simulink model "auv_modell_camsim_vr"  (Simulink 7.0)
settings: Solver=ode45  StartTime=0.0  StopTime=1000  RelTol=1e-3
values from neighbouring files (symbols this model uses):
  eta0 = [-10 -7 7 0 0 0]'    [initauv.m]
undefined symbols (not defined in the file or in its folder): C_calc
libraries: marine_gnc x4, vrlib x2, simulink x1
settings Model: Creator=anderga  LastModifiedBy=anderga  BufferReuse=off
settings OptimizationCC: BlockReduction=off  InlineParams=on  BufferReuse=off

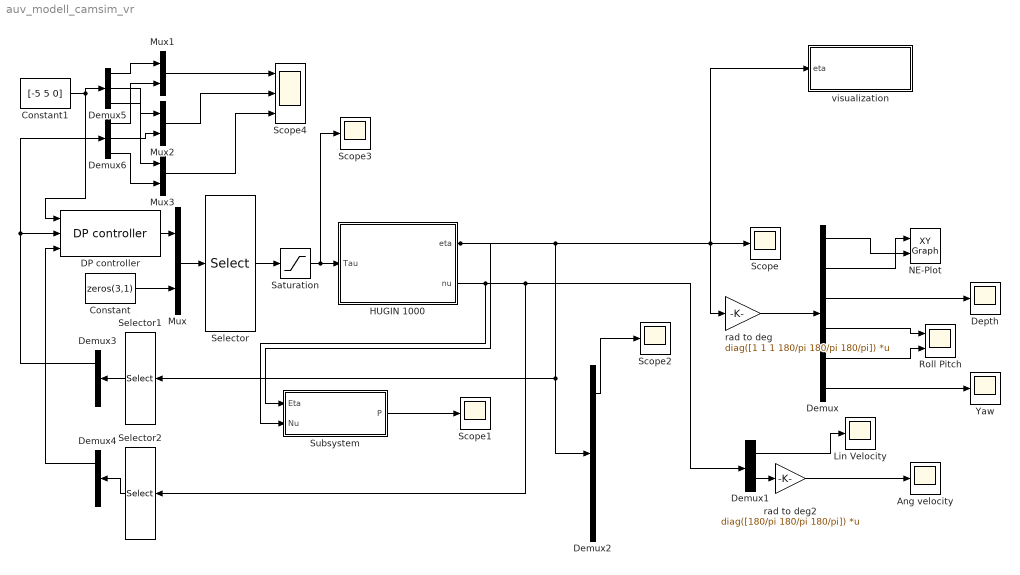
== system auv_modell_camsim_vr ==
  Ang velocity : Scope
      settings: YMin=-0.02  YMax=0.005  SaveName=ScopeData6
  Constant : Constant  Value=zeros(3,1)  OutDataType=sfix(16)  OutScaling=2^0
  Constant1 : Constant  Value=[-5 5 0]  OutDataType=sfix(16)  OutScaling=2^0
  DP controller : marine_gnc/Control/Dynamic  Positioning /DP controller  SystemSampleTime=-1  Kp=diag([230 300 1000])  Kd=diag([750 700 0])  Ki=diag([2 5 0])
  Demux : Demux  Outputs=6
  Demux1 : Demux  Outputs=2
  Demux2 : Demux  Outputs=3
  Demux3 : Demux  Orientation=left  Outputs=2
  Demux4 : Demux  Orientation=left  Outputs=2
  Demux5 : Demux  Outputs=3
  Demux6 : Demux  Outputs=3
  Depth : Scope
      settings: TimeRange=400  YMin=-20  YMax=10  SaveName=ScopeData4
  HUGIN 1000 : Subsystem  mask(HUGIN 1000 AUV){eta_0=eta0, nu_0=[0 0 0 0 0 0]}
      mask prompts: eta_0 "Initial Position [x y z phi theta psi]"; nu_0 "Initial speed [u v w p q r]"
      mask help:
      | The hydrodynamic model of Kongsberg Maritimes
      | AUV type HUGIN 1000.
      |
      | Implemented using
      |
      | eta_dot = J(eta)*nu
      | M*nu_dot + C(nu)*nu + D(nu)*nu + g(eta) = tau
      |
      | and the MMS toolbox from www.marinecybernetics.org
      mask init:
      | m = 1380;
      | xg = 0;
      | yg = 0;
      | zg = 0.0328;
      | Ix = 86.53;
      | Iy = 1247;
      | Iz = 1247;
      | 
      | Xu = -85.57;
      | Yv = -1092.9;
      | Yr = -84.1448;
      | Zw = -1092.9;
      | Zq = 84.1448;
      | Mq = -795.1686;
      | Nr = -795.1686;
      |     
      | M = [m-Xu   0       0       0       m*zg    -m*yg;
      |      0      m-Yv    0       -m*zg   0       m*xg-Yr;
      |      0      0       m-Zw    m*yg    -m*xg-Zq 0;
      |      0      -m*zg   m*yg    Ix      0        0;
      |      m*zg   0       -m*xg-Zq 0      Iy-Mq    0;
      |      -m*yg  m*xg-Yr 0       0       0       Iz-Nr];
  Lin Velocity : Scope
      settings: YMin=-6  YMax=9
  Mux{,1..3} (4 alike) : Mux  Inputs=2
  NE-Plot : simulink/Sinks/XY Graph  SystemSampleTime=-1  xmin=-100  xmax=220  ymin=-100  ymax=100  st=-1
  Roll Pitch : Scope  NumInputPorts=2
      settings: TimeRange=400  YMin=-0.01~-0.015  YMax=0.08~0.015  SaveName=ScopeData3
  Saturation : Saturate  UpperLimit=100  LowerLimit=-100  OutDataType=sfix(16)  OutScaling=2^0
  Scope{,1..3} (4 alike) : Scope
      Scope settings: YMin=-12.5  YMax=7.5
      Scope1 settings: YMin=-1  YMax=1  SaveName=ScopeData9
      Scope2 settings: YMin=-10  YMax=-10  SaveName=ScopeData10
      Scope3 settings: YMin=-100  YMax=100  SaveName=ScopeData11
  Scope4 : Scope  NumInputPorts=3
      settings: YMin=-10~-10~-2.25  YMax=5~12.5~0.75  SaveName=ScopeData12
  Selector : Selector  InputPortWidth=6  IndexOptions=Index vector (dialog)  Indices=[1 2 4 5 6 3]  OutputSizes=1
  Selector1 : Selector  Orientation=left  InputPortWidth=6  IndexOptions=Index vector (dialog)  Indices=[1 2 6 3 4 5]  OutputSizes=1
  Selector2 : Selector  Orientation=left  InputPortWidth=6  IndexOptions=Index vector (dialog)  Indices=[1 2 6 3 4 5]  OutputSizes=1
  Subsystem : Subsystem
  Yaw : Scope
      settings: TimeRange=100  YMin=-27.5  YMax=-7.5  SaveName=ScopeData2
  rad to deg : Gain  Gain=diag([1 1 1 180/pi 180/pi 180/pi])  Multiplication=Matrix(K*u)  ParameterDataType=sfix(16)  ParameterScaling=2^0  OutDataType=sfix(16)  OutScaling=2^0
  rad to deg2 : Gain  Gain=diag([180/pi 180/pi 180/pi])  Multiplication=Matrix(K*u)  ParameterDataType=sfix(16)  ParameterScaling=2^0  OutDataType=sfix(16)  OutScaling=2^0
  visualization : Subsystem
  wires:
  HUGIN 1000/1(eta) -> Subsystem/1(Eta), visualization/1(eta), rad to deg/1, Scope/1, Demux2/1, Selector1/1
  Demux/2 -> NE-Plot/1
  Demux/1 -> NE-Plot/2
  Demux/6 -> Yaw/1
  Demux/4 -> Roll Pitch/1
  Demux/5 -> Roll Pitch/2
  Demux/3 -> Depth/1
  Demux1/1 -> Lin Velocity/1
  Demux1/2 -> rad to deg2/1
  HUGIN 1000/2(nu) -> Subsystem/2(Nu), Demux1/1, Selector2/1
  rad to deg/1 -> Demux/1
  rad to deg2/1 -> Ang velocity/1
  Subsystem/1(P) -> Scope1/1
  Demux2/1 -> Scope2/1
  DP controller/1 -> Mux/1
  Mux/1 -> Selector/1
  Selector/1 -> Saturation/1
  Constant/1 -> Mux/2
  Selector1/1 -> Demux3/1
  Demux3/1 -> DP controller/2, Demux6/1
  Selector2/1 -> Demux4/1
  Demux4/1 -> DP controller/3
  Constant1/1 -> DP controller/1, Demux5/1
  Saturation/1 -> HUGIN 1000/1(Tau), Scope3/1
  Mux1/1 -> Scope4/1
  Mux2/1 -> Scope4/2
  Mux3/1 -> Scope4/3
  Demux5/1 -> Mux1/1
  Demux6/1 -> Mux1/2
  Demux5/2 -> Mux2/1
  Demux5/3 -> Mux3/1
  Demux6/2 -> Mux2/2
  Demux6/3 -> Mux3/2

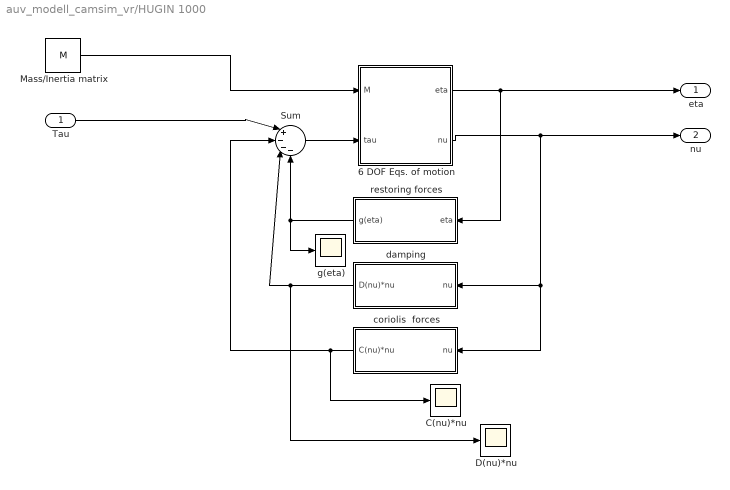
== system auv_modell_camsim_vr/HUGIN 1000 ==
  Tau : Inport  OutDataType=sfix(16)  OutScaling=2^0
  6 DOF Eqs. of motion : Subsystem  AncestorBlock=marine_gnc/Models/ Kinetics /6 DOF Eqs. of motion  mask(Equations of motion){nu0=nu_0, eta0=eta_0}
      mask prompts: nu0 "Initial velocities (u,v,w,p,q,r)"; eta0 "Initial position/attitude (x,y,z,phi,theta,psi)"
      mask help:
      | 6 DOF equations of motion (surge, sway, heave, roll, pitch and yaw)
      |
      |    eta_dot = J(eta)*nu
      |    (M_RB+M_A)*nu_dot  =  tau
      |
      | where nu = [u,v,w,p,q,r]'  and eta = [x,y,z,phi,theta,psi]'
      |
      | T. I. Fossen (2002). Marine Control Systems: Guidance, Navigation and Control of Ships, Rigs and Underwater Vehicles, Marine Cybernetics AS, ISBN 82-92356-00-2
      |
      | Modified by Anders Garmo (2008)
  C(nu)*nu : Scope
      settings: TimeRange=100  YMin=-0.1  YMax=1.2  SaveName=ScopeData5
  D(nu)*nu : Scope
      settings: TimeRange=100  YMin=-10  YMax=100  SaveName=ScopeData8
  Mass/Inertia matrix : Constant  Value=M  OutDataType=sfix(16)  OutScaling=2^0
  Sum : Sum  Inputs=|+---  OutDataType=sfix(16)  OutScaling=2^0
  coriolis  forces : Subsystem  Orientation=left
      mask init:
      | W = 1380*9.81;
      | 
      | zg = 0.0328;
  damping : Subsystem  Orientation=left
      mask init:
      | Xu = -19.1881;
      | Yv = -931.9715;
      | Yr = 1915.8;
      | Zw = -931.9715;
      | Zq = -1915.8;
      | Kp = -1000;
      | Mw = 1760.7;
      | Mq = -8386.3;
      | Nv = -1760.7;
      | Nr = -8386.3;
      | 
      | Xuu = -3.8938;
      | 
      | D = [Xu 0 0 0 0 0;
      |       0 Yv 0 0 0 Yr;
      |       0 0 Zw 0 Zq 0;
      |       0 0 0 Kp 0 0;
      |       0 0 Mw 0 Mq 0;
      |       0 Nv 0 0 0 Nr];
  g(eta) : Scope
      settings: TimeRange=100  YMin=0  YMax=100  SaveName=ScopeData7
  restoring forces : Subsystem  Orientation=left
      mask init:
      | W = 1380*9.81;
      | 
      | zg = 0.0328;
  eta : Outport  OutDataType=sfix(16)  OutScaling=2^0
  nu : Outport  Port=2  OutDataType=sfix(16)  OutScaling=2^0
  wires:
  Mass/Inertia matrix/1 -> 6 DOF Eqs. of motion/1(M)
  6 DOF Eqs. of motion/2(nu) -> nu/1, damping/1(nu), coriolis  forces/1(nu)
  6 DOF Eqs. of motion/1(eta) -> restoring forces/1(eta), eta/1
  Sum/1 -> 6 DOF Eqs. of motion/2(tau)
  Tau/1 -> Sum/1
  coriolis  forces/1(C(nu)*nu) -> C(nu)*nu/1, Sum/2
  restoring forces/1(g(eta)) -> Sum/4, g(eta)/1
  damping/1(D(nu)*nu) -> Sum/3, D(nu)*nu/1

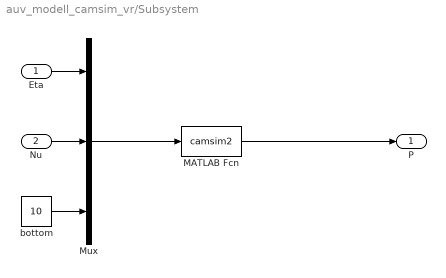
== system auv_modell_camsim_vr/Subsystem ==
  Eta : Inport  OutDataType=sfix(16)  OutScaling=2^0
  Nu : Inport  Port=2  OutDataType=sfix(16)  OutScaling=2^0
  MATLAB Fcn : MATLABFcn  MATLABFcn=camsim2  OutputDimensions=6
  Mux : Mux  Inputs=3
  bottom : Constant  Value=10  OutDataType=sfix(16)  OutScaling=2^0
  P : Outport  OutDataType=sfix(16)  OutScaling=2^0
  wires:
  Eta/1 -> Mux/1
  Nu/1 -> Mux/2
  bottom/1 -> Mux/3
  Mux/1 -> MATLAB Fcn/1
  MATLAB Fcn/1 -> P/1

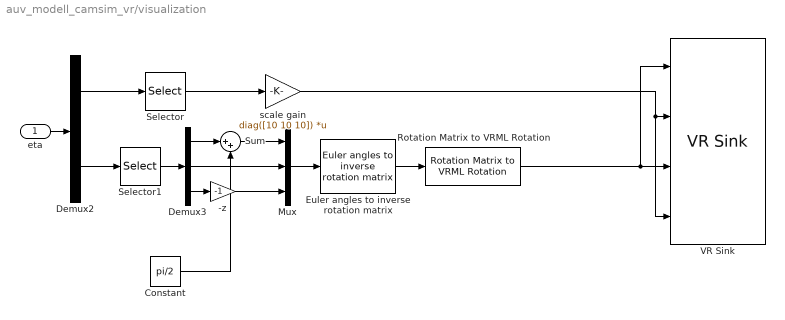
== system auv_modell_camsim_vr/visualization ==
  eta : Inport  OutDataType=sfix(16)  OutScaling=2^0
  -z : Gain  Gain=-1  ParameterDataType=sfix(16)  ParameterScaling=2^0  OutDataType=sfix(16)  OutScaling=2^0
  Constant : Constant  Value=pi/2  OutDataType=sfix(16)  OutScaling=2^0
  Demux2 : Demux  Outputs=2
  Demux3 : Demux  Outputs=3
  Euler angles to inverse rotation matrix : marine_gnc/Models/ Kinematics/Euler angles to inverse rotation matrix  SystemSampleTime=-1
  Mux : Mux  Inputs=3
  Rotation Matrix to VRML Rotation : vrlib/Utilities/Rotation Matrix to VRML Rotation  SystemSampleTime=-1  maxzero=1e-12
  Selector : Selector  InputPortWidth=3  IndexOptions=Index vector (dialog)  Indices=[2 3 1]  OutputSizes=1
  Selector1 : Selector  InputPortWidth=3  IndexOptions=Index vector (dialog)  Indices=[2 1 3]  OutputSizes=1
  Sum : Sum  Inputs=|++  OutDataType=sfix(16)  OutScaling=2^0
  VR Sink : vrlib/VR Sink  SampleTime=0.1  ViewEnable=on  RemoteChange=off  RemoteView=off  FieldsWritten=Mounted.orientation.4.1.double#Mounted.position.3.1.double#Hugin1000.rotation.4.1.double#Hugin1000.translation.3.1.double  WorldFileName=M:\tex\svn\3d-modell\hugin.WRL  AutoView=on  VideoDimensions=[]  FigureProperties="{'Position', 'Name', 'Viewpoint', 'CameraBound', 'CameraDirection', 'CameraPosition', 'CameraUpVector', 'ZoomFactor', 'Antialiasing', 'Headlight', 'Lighting', 'NavPanel', 'StatusBar', 'ToolBar', 'Textures', 'Transparency', 'Wireframe', 'NavZones', 'NavMode', 'NavSpeed', 'Record2DCompressMethod', 'Record2DCompressQuality', 'Record2D', 'Record2DFileName', 'Record2DFPS'; [8.0000000000000000e+000  8.6000000000000000e+001  6.2600000000000000e+002  4.0100000000000000e+002], '', 'Overview', 'on', [-4.7477468383467128e-002 -4.8324566214636475e-002 -9.9770267429534354e-001], [2.2305288483536316e+001  9.0696940792763357e+001  3.7396872559245497e+002], [-5.7495926579068657e-003  9.9882571893031757e-001 -4.8105357161235845e-002], [1.0000000000000000e+000], 'off', 'on', 'on', 'halfbar', 'off', 'on', 'on', 'on', 'off', 'off', 'walk', 'normal', 'auto', [7.5000000000000000e+001], 'off', '%f_anim_%n.avi', [1.5000000000000000e+001]}"
  scale gain : Gain  Gain=diag([10 10 10])  Multiplication=Matrix(K*u)  ParameterDataType=sfix(16)  ParameterScaling=2^0  OutDataType=sfix(16)  OutScaling=2^0
  wires:
  Demux2/1 -> Selector/1
  Selector/1 -> scale gain/1
  Euler angles to inverse rotation matrix/1 -> Rotation Matrix to VRML Rotation/1
  Demux2/2 -> Selector1/1
  Selector1/1 -> Demux3/1
  Mux/1 -> Euler angles to inverse rotation matrix/1
  Demux3/3 -> -z/1
  Constant/1 -> Sum/2
  Demux3/1 -> Sum/1
  Sum/1 -> Mux/1
  Demux3/2 -> Mux/2
  -z/1 -> Mux/3
  eta/1 -> Demux2/1
  Rotation Matrix to VRML Rotation/1 -> VR Sink/3, VR Sink/1
  scale gain/1 -> VR Sink/2, VR Sink/4

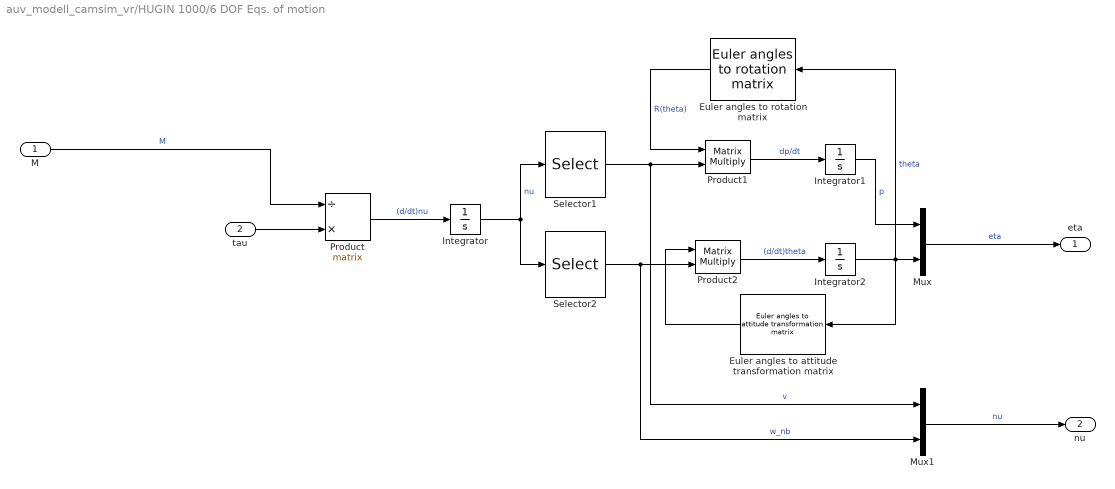
== system auv_modell_camsim_vr/HUGIN 1000/6 DOF Eqs. of motion ==
  M : Inport  OutDataType=sfix(16)  OutScaling=2^0
  tau : Inport  Port=2  OutDataType=sfix(16)  OutScaling=2^0
  Euler angles to rotation matrix : marine_gnc/Models/ Kinematics/Euler angles to rotation matrix  Orientation=left  SystemSampleTime=-1
  Euler angles to attitude transformation matrix : marine_gnc/Models/ Kinematics/Euler angles to attitude transformation matrix  Orientation=left  SystemSampleTime=-1
  Integrator : Integrator  InitialCondition=nu0
  Integrator1 : Integrator  InitialCondition=eta0(1:3)
  Integrator2 : Integrator  InitialCondition=eta0(4:6)
  Mux : Mux  Inputs=2
  Mux1 : Mux  Inputs=2
  Product : Product  Inputs=/*  Multiplication=Matrix(*)  OutDataType=sfix(16)  OutScaling=2^0  SaturateOnIntegerOverflow=on
  Product1 : Product  Inputs=**  Multiplication=Matrix(*)  OutDataType=sfix(16)  OutScaling=2^0  SaturateOnIntegerOverflow=on
  Product2 : Product  Inputs=**  Multiplication=Matrix(*)  OutDataType=sfix(16)  OutScaling=2^0  SaturateOnIntegerOverflow=on
  Selector1 : Selector  InputPortWidth=6  IndexOptions=Index vector (dialog)  Indices=[1 2 3]  OutputSizes=1
  Selector2 : Selector  InputPortWidth=6  IndexOptions=Index vector (dialog)  Indices=[4 5 6]  OutputSizes=1
  eta : Outport  OutDataType=sfix(16)  OutScaling=2^0
  nu : Outport  Port=2  OutDataType=sfix(16)  OutScaling=2^0
  wires:
  tau/1 -> Product/2
  Euler angles to attitude transformation matrix/1 -> Product2/1
  Mux1/1 -> nu/1  "nu"
  Mux/1 -> eta/1  "eta"
  Integrator1/1 -> Mux/1  "p"
  Integrator2/1 -> Euler angles to attitude transformation matrix/1, Euler angles to rotation matrix/1, Mux/2  "theta"
  Product2/1 -> Integrator2/1  "(d/dt)theta"
  Euler angles to rotation matrix/1 -> Product1/1  "R(theta)"
  Product1/1 -> Integrator1/1  "dp/dt"
  Selector2/1 -> Product2/2, Mux1/2  "w_nb"
  Selector1/1 -> Mux1/1, Product1/2  "v"
  Integrator/1 -> Selector2/1, Selector1/1  "nu"
  Product/1 -> Integrator/1  "(d/dt)nu"
  M/1 -> Product/1  "M"

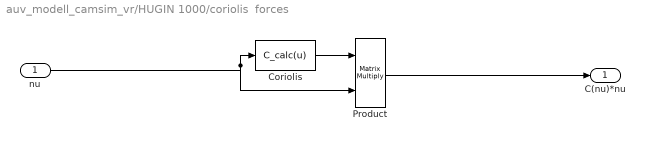
== system auv_modell_camsim_vr/HUGIN 1000/coriolis  forces ==
  nu : Inport  OutDataType=sfix(16)  OutScaling=2^0
  Coriolis : MATLABFcn  MATLABFcn=C_calc(u)  OutputDimensions=[6,6]  Output1D=off
  Product : Product  Multiplication=Matrix(*)  OutDataType=sfix(16)  OutScaling=2^0  RndMeth=Zero
  C(nu)*nu : Outport  OutDataType=sfix(16)  OutScaling=2^0
  wires:
  nu/1 -> Product/2, Coriolis/1
  Coriolis/1 -> Product/1
  Product/1 -> C(nu)*nu/1

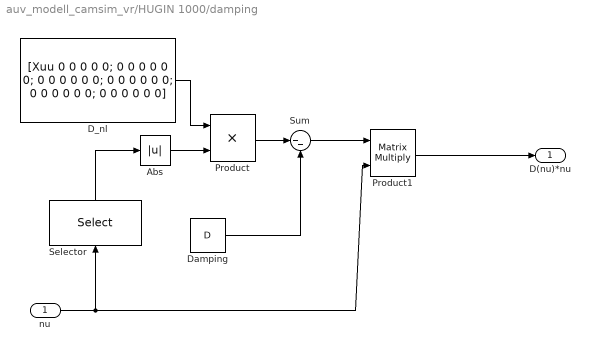
== system auv_modell_camsim_vr/HUGIN 1000/damping ==
  nu : Inport  OutDataType=sfix(16)  OutScaling=2^0
  Abs : Abs  OutDataType=sfix(16)  OutScaling=2^0
  D_nl : Constant  Value=[Xuu 0 0 0 0 0; 0 0 0 0 0 0; 0 0 0 0 0 0; 0 0 0 0 0 0; 0 0 0 0 0 0; 0 0 0 0 0 0]  OutDataType=sfix(16)  OutScaling=2^0
  Damping : Constant  Value=D  OutDataType=sfix(16)  OutScaling=2^0
  Product : Product  OutDataType=sfix(16)  OutScaling=2^0  RndMeth=Zero
  Product1 : Product  Multiplication=Matrix(*)  OutDataType=sfix(16)  OutScaling=2^0  RndMeth=Zero
  Selector : Selector  Orientation=up  InputPortWidth=6  IndexOptions=Index vector (dialog)  Indices=[1]  OutputSizes=1
  Sum : Sum  Inputs=|--  OutDataType=sfix(16)  OutScaling=2^0
  D(nu)*nu : Outport  OutDataType=sfix(16)  OutScaling=2^0
  wires:
  Damping/1 -> Sum/2
  Product/1 -> Sum/1
  nu/1 -> Product1/2, Selector/1
  D_nl/1 -> Product/1
  Abs/1 -> Product/2
  Sum/1 -> Product1/1
  Product1/1 -> D(nu)*nu/1
  Selector/1 -> Abs/1

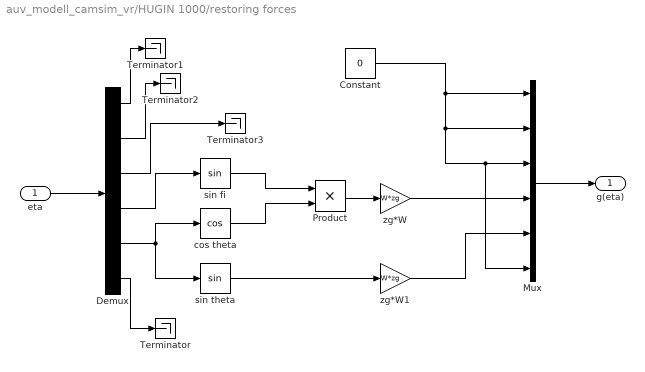
== system auv_modell_camsim_vr/HUGIN 1000/restoring forces ==
  eta : Inport  OutDataType=sfix(16)  OutScaling=2^0
  Constant : Constant  Value=0  OutDataType=sfix(16)  OutScaling=2^0
  Demux : Demux  Outputs=6
  Mux : Mux  Inputs=6
  Product : Product  OutDataType=sfix(16)  OutScaling=2^0  RndMeth=Zero
  Terminator{,1..3} (4 alike) : Terminator
  cos theta : Trigonometry  Operator=cos
  sin fi : Trigonometry
  sin theta : Trigonometry
  zg*W : Gain  Gain=W*zg  ParameterDataType=sfix(16)  ParameterScaling=2^0  OutDataType=sfix(16)  OutScaling=2^0
  zg*W1 : Gain  Gain=W*zg  ParameterDataType=sfix(16)  ParameterScaling=2^0  OutDataType=sfix(16)  OutScaling=2^0
  g(eta) : Outport  OutDataType=sfix(16)  OutScaling=2^0
  wires:
  eta/1 -> Demux/1
  Demux/4 -> sin fi/1
  Demux/5 -> cos theta/1, sin theta/1
  cos theta/1 -> Product/2
  sin fi/1 -> Product/1
  Product/1 -> zg*W/1
  sin theta/1 -> zg*W1/1
  Mux/1 -> g(eta)/1
  zg*W1/1 -> Mux/5
  zg*W/1 -> Mux/4
  Constant/1 -> Mux/1, Mux/2, Mux/3, Mux/6
  Demux/6 -> Terminator/1
  Demux/1 -> Terminator1/1
  Demux/2 -> Terminator2/1
  Demux/3 -> Terminator3/1
